simulink model "TSR_Scenario_003_cs"  (R2014b)
settings: Solver=ode5  SolverMode=SingleTasking  StartTime=0.0  StopTime=inf  FixedStep=1/100  RelTol=1e-3
PreLoadFcn:
  | mbxruntime.callbacks.PreLoadFcn(bdroot);
  | check_NUTS_defined;
  | 
  | assignin('base',['model_closed_' bdroot],false);
  | 
  | addpath('../includes_TSR/includes_TSR');
  | 
  | switch version('-release')
  | case {'2010a', '2010b', '2011a'}
  | addpath('../includes_TSR/ML2010b');
  | otherwise
  | addpath('../includes_TSR/ML2011b');
  | end
PostLoadFcn:
  | mbxruntime.callbacks.PostLoadFcn(bdroot);
InitFcn:
  | mbxruntime.callbacks.InitFcn(bdroot);
StartFcn:
  | mbxruntime.callbacks.StartFcn(bdroot);
StopFcn:
  | mbxruntime.callbacks.StopFcn(bdroot);
model workspace: external: MAT-File .\TSR_Scenario_003_cs_hws.mat (data not in the file)
undefined symbols (not defined in the file or in its folder): InitImageOutputDir, mbxruntime, OrientationPitch, OrientationRoll, PositionX, PositionY, PositionZ, tabledata, warningInitialVelocity, x0
undefined symbols (not defined in the file): SteeringColumn, SteeringWheel, TSR_Scenario_003_cs_031c08980fc50484, TSR_Scenario_003_cs_034f292ed02288d5, TSR_Scenario_003_cs_0459b3dfbc82c9a8, TSR_Scenario_003_cs_097620f815f21f1d, TSR_Scenario_003_cs_097d7573cc694bf5, TSR_Scenario_003_cs_0996a1a3dd5e2a3a, TSR_Scenario_003_cs_0f1849cdb4701326, TSR_Scenario_003_cs_10f4098912b3b5db, TSR_Scenario_003_cs_117f01ea831ec368, TSR_Scenario_003_cs_12cf78b79d36da1c, TSR_Scenario_003_cs_144fbb977118bf37, TSR_Scenario_003_cs_1523d5367c5052d0, TSR_Scenario_003_cs_1540f37e1ce5220e, TSR_Scenario_003_cs_15da4682074a9114, TSR_Scenario_003_cs_186e86d78e8adde8, TSR_Scenario_003_cs_198fefcb5c5d4c4a, TSR_Scenario_003_cs_1d24564a28ca8c57, TSR_Scenario_003_cs_1ea9b65b93b2d93e, TSR_Scenario_003_cs_1f4a4c0163bc654f, TSR_Scenario_003_cs_221c7f4f757b6f59, TSR_Scenario_003_cs_22229c9f69845439, TSR_Scenario_003_cs_230bf92302b3240a, TSR_Scenario_003_cs_23763ac742803108, TSR_Scenario_003_cs_237ee3c37f4d72b6, TSR_Scenario_003_cs_2956d712ba1268bc, TSR_Scenario_003_cs_2c8e6bdc42e74688, TSR_Scenario_003_cs_3037724928f99df0, TSR_Scenario_003_cs_31b44ca47ec5ff02, TSR_Scenario_003_cs_324745b613f45b9c, TSR_Scenario_003_cs_32b36e3fd4699b17, TSR_Scenario_003_cs_35d6077a5f3bdf8f, TSR_Scenario_003_cs_364710b5c901cafc, TSR_Scenario_003_cs_3727ee2f4430f2bb, TSR_Scenario_003_cs_382e41ab6806a13f, TSR_Scenario_003_cs_38ccddae174883be, TSR_Scenario_003_cs_3a0767dbf486e31b, TSR_Scenario_003_cs_3b460d19c10c747b, TSR_Scenario_003_cs_426c63b9f9c7abdf, TSR_Scenario_003_cs_42f1edf1b324bf4e, TSR_Scenario_003_cs_43b33e682c00a164, TSR_Scenario_003_cs_440a2f0d77aab01b, TSR_Scenario_003_cs_466378c5e179d625, TSR_Scenario_003_cs_4b8aa743d5bd8c1e, TSR_Scenario_003_cs_4bb095d5f4984042, TSR_Scenario_003_cs_4cec1a92176fe53d, TSR_Scenario_003_cs_4d6b6c843c52af2c, TSR_Scenario_003_cs_514fc139d324fd0d, TSR_Scenario_003_cs_51f4eff9e91179f9, TSR_Scenario_003_cs_56a9ea09cd860a89, TSR_Scenario_003_cs_5749c15298076949, TSR_Scenario_003_cs_576a8029b2a2792f, TSR_Scenario_003_cs_58b2f104991e8ca9, TSR_Scenario_003_cs_59a8a0af3bc025d5, TSR_Scenario_003_cs_5baf0e640050f43b, TSR_Scenario_003_cs_626299c795c4a86e, TSR_Scenario_003_cs_6499aa317499632d, TSR_Scenario_003_cs_676e881463a7df3e, TSR_Scenario_003_cs_68379cf1a8816ef6 ... (+115)
libraries: PreScanSimulinkLibrary x53, simulink_extras x37, simulink x29
(part 10 of 21)

== system TSR_Scenario_003_cs/Audi_A8_1/SteeringColumn_pivot_Mux ==
  X [m] : Inport
  Y [m] : Inport  Port=2
  Z [m] : Inport  Port=3
  Roll [rad] : Inport  Port=4
  Pitch [rad] : Inport  Port=5
  Yaw [rad] : Inport  Port=6
  Bus Creator : BusCreator  Inputs=3  OutDataTypeStr=Bus: PRESCAN_XYZ_DATA
  Bus Creator1 : BusCreator  Inputs=3  OutDataTypeStr=Bus: PRESCAN_RPY_DATA
  Bus Creator2 : BusCreator  Inputs=2  OutDataTypeStr=Bus: PRESCAN_POSE_DATA
  Joint : Outport
  wires:
  Yaw [rad]/1 -> Bus Creator1/3  "Yaw"
  Bus Creator1/1 -> Bus Creator2/2  "ORIENTATION"
  Bus Creator/1 -> Bus Creator2/1  "POSITION"
  X [m]/1 -> Bus Creator/1  "X"
  Y [m]/1 -> Bus Creator/2  "Y"
  Z [m]/1 -> Bus Creator/3  "Z"
  Bus Creator2/1 -> Joint/1
  Roll [rad]/1 -> Bus Creator1/1  "Roll"
  Pitch [rad]/1 -> Bus Creator1/2  "Pitch"

== system TSR_Scenario_003_cs/Audi_A8_1/SteeringWheel_pivot_Mux ==
  X [m] : Inport
  Y [m] : Inport  Port=2
  Z [m] : Inport  Port=3
  Roll [rad] : Inport  Port=4
  Pitch [rad] : Inport  Port=5
  Yaw [rad] : Inport  Port=6
  Bus Creator : BusCreator  Inputs=3  OutDataTypeStr=Bus: PRESCAN_XYZ_DATA
  Bus Creator1 : BusCreator  Inputs=3  OutDataTypeStr=Bus: PRESCAN_RPY_DATA
  Bus Creator2 : BusCreator  Inputs=2  OutDataTypeStr=Bus: PRESCAN_POSE_DATA
  Joint : Outport
  wires:
  Yaw [rad]/1 -> Bus Creator1/3  "Yaw"
  Bus Creator1/1 -> Bus Creator2/2  "ORIENTATION"
  Bus Creator/1 -> Bus Creator2/1  "POSITION"
  X [m]/1 -> Bus Creator/1  "X"
  Y [m]/1 -> Bus Creator/2  "Y"
  Z [m]/1 -> Bus Creator/3  "Z"
  Bus Creator2/1 -> Joint/1
  Roll [rad]/1 -> Bus Creator1/1  "Roll"
  Pitch [rad]/1 -> Bus Creator1/2  "Pitch"

== system TSR_Scenario_003_cs/Audi_A8_1/WheelDisplacement_Mux ==
  Steering Angle Front [rad] : Inport  Tag=inport/JointGroup  SampleTime=1/100  BusOutputAsStruct=on
  Steering Angle Rear [rad] : Inport  Tag=inport/JointGroup  Port=2  SampleTime=1/100  BusOutputAsStruct=on
  Rotation [rad] : Inport  Tag=inport/JointGroup  Port=3  SampleTime=1/100  BusOutputAsStruct=on
  zDisp FL [m] : Inport  Tag=inport/JointGroup  Port=4  SampleTime=1/100  BusOutputAsStruct=on
  zDisp FR [m] : Inport  Tag=inport/JointGroup  Port=5  SampleTime=1/100  BusOutputAsStruct=on
  zDisp RL [m] : Inport  Tag=inport/JointGroup  Port=6  SampleTime=1/100  BusOutputAsStruct=on
  zDisp RR [m] : Inport  Tag=inport/JointGroup  Port=7  SampleTime=1/100  BusOutputAsStruct=on
  Ground_{1..12} (12 alike) : Ground
  WheelL0_Mux : Subsystem  Tag=mux/Joint  mask(PreScan Mux Block){DisplayName=WheelL0}
      mask prompts: DisplayName "Display Name"
      mask help:
      | This block simulates a generic joint used for generic models. This joint can be enabled/disabled from the GUI.
      |
      | For more information, please click Help.
      settings: DeleteFcn=PreScanBlockDeleteFcn;
      mask Help: eval('openHelp(254)')
  WheelL1_Mux : Subsystem  Tag=mux/Joint  mask(PreScan Mux Block){DisplayName=WheelL1}
      mask prompts: DisplayName "Display Name"
      mask help:
      | This block simulates a generic joint used for generic models. This joint can be enabled/disabled from the GUI.
      |
      | For more information, please click Help.
      settings: DeleteFcn=PreScanBlockDeleteFcn;
      mask Help: eval('openHelp(254)')
  WheelR0_Mux : Subsystem  Tag=mux/Joint  mask(PreScan Mux Block){DisplayName=WheelR0}
      mask prompts: DisplayName "Display Name"
      mask help:
      | This block simulates a generic joint used for generic models. This joint can be enabled/disabled from the GUI.
      |
      | For more information, please click Help.
      settings: DeleteFcn=PreScanBlockDeleteFcn;
      mask Help: eval('openHelp(254)')
  WheelR1_Mux : Subsystem  Tag=mux/Joint  mask(PreScan Mux Block){DisplayName=WheelR1}
      mask prompts: DisplayName "Display Name"
      mask help:
      | This block simulates a generic joint used for generic models. This joint can be enabled/disabled from the GUI.
      |
      | For more information, please click Help.
      settings: DeleteFcn=PreScanBlockDeleteFcn;
      mask Help: eval('openHelp(254)')
  WheelL0_Audi_A8_1 : Outport  Tag=outport/JointActuator  OutDataTypeStr=Bus: PRESCAN_POSE_DATA  SampleTime=1/100
  WheelL1_Audi_A8_1 : Outport  Tag=outport/JointActuator  Port=2  OutDataTypeStr=Bus: PRESCAN_POSE_DATA  SampleTime=1/100
  WheelR0_Audi_A8_1 : Outport  Tag=outport/JointActuator  Port=3  OutDataTypeStr=Bus: PRESCAN_POSE_DATA  SampleTime=1/100
  WheelR1_Audi_A8_1 : Outport  Tag=outport/JointActuator  Port=4  OutDataTypeStr=Bus: PRESCAN_POSE_DATA  SampleTime=1/100
  wires:
  WheelL0_Mux/1(Joint) -> WheelL0_Audi_A8_1/1
  WheelL1_Mux/1(Joint) -> WheelL1_Audi_A8_1/1
  WheelR0_Mux/1(Joint) -> WheelR0_Audi_A8_1/1
  WheelR1_Mux/1(Joint) -> WheelR1_Audi_A8_1/1
  Steering Angle Front [rad]/1 -> WheelR0_Mux/6(Yaw [rad]), WheelL0_Mux/6(Yaw [rad])
  Steering Angle Rear [rad]/1 -> WheelR1_Mux/6(Yaw [rad]), WheelL1_Mux/6(Yaw [rad])
  Rotation [rad]/1 -> WheelR0_Mux/5(Pitch [rad]), WheelL0_Mux/5(Pitch [rad]), WheelR1_Mux/5(Pitch [rad]), WheelL1_Mux/5(Pitch [rad])
  zDisp FL [m]/1 -> WheelL0_Mux/3(Z [m])
  zDisp FR [m]/1 -> WheelR0_Mux/3(Z [m])
  zDisp RL [m]/1 -> WheelL1_Mux/3(Z [m])
  zDisp RR [m]/1 -> WheelR1_Mux/3(Z [m])
  Ground_1/1 -> WheelL0_Mux/1(X [m])
  Ground_2/1 -> WheelL0_Mux/2(Y [m])
  Ground_3/1 -> WheelL0_Mux/4(Roll [rad])
  Ground_4/1 -> WheelL1_Mux/1(X [m])
  Ground_5/1 -> WheelL1_Mux/2(Y [m])
  Ground_6/1 -> WheelL1_Mux/4(Roll [rad])
  Ground_7/1 -> WheelR0_Mux/1(X [m])
  Ground_8/1 -> WheelR0_Mux/2(Y [m])
  Ground_9/1 -> WheelR0_Mux/4(Roll [rad])
  Ground_10/1 -> WheelR1_Mux/1(X [m])
  Ground_11/1 -> WheelR1_Mux/2(Y [m])
  Ground_12/1 -> WheelR1_Mux/4(Roll [rad])

== system TSR_Scenario_003_cs/Audi_A8_1/d2r SteeringColumn_pivot_Mux ==
  Degrees in : Inport
  Gain1 : Gain  Gain=pi/180  SaturateOnIntegerOverflow=on  OutDataTypeStr=Inherit: Same as input  ParamDataTypeStr=Inherit: Same as input
  Radians out : Outport  InitialOutput=0
  wires:
  Gain1/1 -> Radians out/1
  Degrees in/1 -> Gain1/1

== system TSR_Scenario_003_cs/Audi_A8_1/d2r SteeringWheel_pivot_Mux ==
  Degrees in : Inport
  Gain1 : Gain  Gain=pi/180  SaturateOnIntegerOverflow=on  OutDataTypeStr=Inherit: Same as input  ParamDataTypeStr=Inherit: Same as input
  Radians out : Outport  InitialOutput=0
  wires:
  Gain1/1 -> Radians out/1
  Degrees in/1 -> Gain1/1

== system TSR_Scenario_003_cs/Audi_A8_1/d2r WheelDisplacement_Mux 1 ==
  Degrees in : Inport
  Gain1 : Gain  Gain=pi/180  SaturateOnIntegerOverflow=on  OutDataTypeStr=Inherit: Same as input  ParamDataTypeStr=Inherit: Same as input
  Radians out : Outport  InitialOutput=0
  wires:
  Gain1/1 -> Radians out/1
  Degrees in/1 -> Gain1/1

== system TSR_Scenario_003_cs/BMW_X5_1/Dynamics_Empty ==
  note: For state mode 'Dynamic' positions
      | are not taken into account, as they
      | are computed by integrating velocity.
      | Click annotation for Help.
  note: For state mode 'Dynamic' positions
      | are not taken into account, as they
      | are computed by integrating velocity.
      | Click annotation for Help.
  Ground_{1..9} (9 alike) : Ground
  MuxState : Subsystem  Tag=mux/State  mask(Empty Dynamics State Block){positioningmode=on, TimeStep=1/100}
      mask prompts: positioningmode "Positioning Mode"; TimeStep "Auto Assigned: Time Step [s]"
      mask help:
      | Build the state of an actor based on user input.
      | The user can either use positioning mode or dynamics mode.
      | - When using positioning mode the position and orientation of the actor are set directly based on the input. Expected input is relative to the initial position and orientation of the actor. It's also possible to specify the velocity of the actor, though this input isn't used, only passed on.
      | - When using dynamics mode the position input is ignored. Expected input is velocity and orientation. The velocity is relative the current orientation of the actor, while orientation is relative to its initial orientation. The position of the actor is calculated based on the velocity and orientation given.
      settings: DeleteFcn=PreScanBlockDeleteFcn;
  STATE_BMW_X5_1 : Subsystem  Tag=mux/StatePort  Priority=0  LoadFcn=load PrescanStateActuatorData  mask(PreScan Sink Block: State){x0=TSR_Scenario_003_cs_BMW_X5_1_Dynamics_Empty_STATE_BMW_X5_1_x0, y0=TSR_Scenario_003_cs_BMW_X5_1_Dynamics_Empty_STATE_BMW_X5_1_y0, z0=TSR_Scenario_003_cs_BMW_X5_1_Dynamics_Empty_STATE_BMW_X5_1_z0, Roll0=TSR_Scenario_003_cs_15da4682074a9114, Pitch0=TSR_Scenario_003_cs_d01058e0ce79997b, Yaw0=TSR_Scenario_003_cs_BMW_X5_1_Dynamics_Empty_STATE_BMW_X5_1_Yaw0, TimeStep=1/100}
      mask prompts: x0 "Ini x-position VEHICLE wrt GLOBAL axis system [m]"; y0 "Ini y-position VEHICLE wrt GLOBAL axis system [m]"; z0 "Ini z-position VEHICLE wrt GLOBAL axis system [m]"; Roll0 "Ini roll-angle BODY wrt VEHICLE axis system [deg]"; Pitch0 "Ini pitch-angle BODY wrt VEHICLE axis system [deg]"; Yaw0 "Ini yaw-angle VEHICLE wrt GLOBAL axis system [deg]"; TimeStep "Auto-Assigned: Upload Period [s]"
      mask help:
      | The Actor State contains a vector signal of size (9x1), containing the following signals:
      |
      | -  Position                  (x,y,z)                                     [m]
      | -  Velocity                  (vx,vy,vz)                               [m/s]
      | -  Angles                    (Roll, Pitch, Yaw)                   [rad]
      |
      | The Actor state is defined in the global axis system.
      | The state is superponed on the Initial position defined in the GUI.
      |
      | For more information, please click Help.
      settings: DeleteFcn=PreScanBlockDeleteFcn;
      mask Help: eval('openHelp(222)')
      mask Display: image(imread('State.png'))
  State : Outport  Tag=outport/StateOutport  SampleTime=1/100
  wires:
  STATE_BMW_X5_1/1(StateBus) -> State/1
  MuxState/1(state) -> STATE_BMW_X5_1/1(State)
  Ground_1/1 -> MuxState/1(x [m])
  Ground_2/1 -> MuxState/2(y [m])
  Ground_3/1 -> MuxState/3(z [m])
  Ground_4/1 -> MuxState/4(dx [m/s])
  Ground_5/1 -> MuxState/5(dy [m/s])
  Ground_6/1 -> MuxState/6(dz [m/s])
  Ground_7/1 -> MuxState/7(R [rad])
  Ground_8/1 -> MuxState/8(P [rad])
  Ground_9/1 -> MuxState/9(Y [rad])

== system TSR_Scenario_003_cs/BMW_X5_1/SELF_Demux ==
  SELF : Inport  OutDataTypeStr=Bus: PRESCAN_SELFSENSORDATA
  Bus Selector : BusSelector  OutputSignals=PositionX,PositionY,PositionZ,OrientationRoll,OrientationPitch,OrientationYaw,Velocity,Yaw_rate,Lat,Long,Alt
  Demux2 : Demux  Outputs=3
  Gain : Gain  Gain=180/pi
  Gain1 : Gain  Gain=180/pi
  Vector Concatenate1 : Concatenate  NumInputs=3
  compas converter : Subsystem
  x [m] : Outport
  y [m] : Outport  Port=2
  z [m] : Outport  Port=3
  rotx [deg] : Outport  Port=4
  roty [deg] : Outport  Port=5
  rotz [deg] : Outport  Port=6
  GPS lat [deg] : Outport  Port=7
  GPS long [deg] : Outport  Port=8
  GPS alt [m] : Outport  Port=9
  velocity [m/s] : Outport  Port=10
  heading [deg] : Outport  Port=11
  yaw rate [deg/s] : Outport  Port=12
  wires:
  Bus Selector/11 -> GPS alt [m]/1  "<Alt>"
  Bus Selector/10 -> GPS long [deg]/1  "<Long>"
  Bus Selector/9 -> GPS lat [deg]/1  "<Lat>"
  Bus Selector/8 -> Gain1/1  "<Yaw_rate>"
  Bus Selector/7 -> velocity [m/s]/1  "<Velocity>"
  Bus Selector/6 -> compas converter/1(rotz [rad]), Vector Concatenate1/3  "<OrientationYaw>"
  Bus Selector/5 -> Vector Concatenate1/2  "<OrientationPitch>"
  Bus Selector/4 -> Vector Concatenate1/1  "<OrientationRoll>"
  Vector Concatenate1/1 -> Gain/1
  Bus Selector/3 -> z [m]/1  "<PositionZ>"
  Bus Selector/2 -> y [m]/1  "<PositionY>"
  Bus Selector/1 -> x [m]/1  "<PositionX>"
  SELF/1 -> Bus Selector/1
  Gain/1 -> Demux2/1
  Demux2/1 -> rotx [deg]/1
  Demux2/2 -> roty [deg]/1
  Demux2/3 -> rotz [deg]/1
  compas converter/1(heading [deg]) -> heading [deg]/1
  Gain1/1 -> yaw rate [deg/s]/1

== system TSR_Scenario_003_cs/BMW_X5_2/Dynamics_Empty ==
  note: For state mode 'Dynamic' positions
      | are not taken into account, as they
      | are computed by integrating velocity.
      | Click annotation for Help.
  note: For state mode 'Dynamic' positions
      | are not taken into account, as they
      | are computed by integrating velocity.
      | Click annotation for Help.
  Ground_{1..9} (9 alike) : Ground
  MuxState : Subsystem  Tag=mux/State  mask(Empty Dynamics State Block){positioningmode=on, TimeStep=1/100}
      mask prompts: positioningmode "Positioning Mode"; TimeStep "Auto Assigned: Time Step [s]"
      mask help:
      | Build the state of an actor based on user input.
      | The user can either use positioning mode or dynamics mode.
      | - When using positioning mode the position and orientation of the actor are set directly based on the input. Expected input is relative to the initial position and orientation of the actor. It's also possible to specify the velocity of the actor, though this input isn't used, only passed on.
      | - When using dynamics mode the position input is ignored. Expected input is velocity and orientation. The velocity is relative the current orientation of the actor, while orientation is relative to its initial orientation. The position of the actor is calculated based on the velocity and orientation given.
      settings: DeleteFcn=PreScanBlockDeleteFcn;
  STATE_BMW_X5_2 : Subsystem  Tag=mux/StatePort  Priority=0  LoadFcn=load PrescanStateActuatorData  mask(PreScan Sink Block: State){x0=TSR_Scenario_003_cs_BMW_X5_2_Dynamics_Empty_STATE_BMW_X5_2_x0, y0=TSR_Scenario_003_cs_BMW_X5_2_Dynamics_Empty_STATE_BMW_X5_2_y0, z0=TSR_Scenario_003_cs_BMW_X5_2_Dynamics_Empty_STATE_BMW_X5_2_z0, Roll0=TSR_Scenario_003_cs_683e8ba4a0f8240e, Pitch0=TSR_Scenario_003_cs_bee4b2d4b9008bb0, Yaw0=TSR_Scenario_003_cs_BMW_X5_2_Dynamics_Empty_STATE_BMW_X5_2_Yaw0, TimeStep=1/100}
      mask prompts: x0 "Ini x-position VEHICLE wrt GLOBAL axis system [m]"; y0 "Ini y-position VEHICLE wrt GLOBAL axis system [m]"; z0 "Ini z-position VEHICLE wrt GLOBAL axis system [m]"; Roll0 "Ini roll-angle BODY wrt VEHICLE axis system [deg]"; Pitch0 "Ini pitch-angle BODY wrt VEHICLE axis system [deg]"; Yaw0 "Ini yaw-angle VEHICLE wrt GLOBAL axis system [deg]"; TimeStep "Auto-Assigned: Upload Period [s]"
      mask help:
      | The Actor State contains a vector signal of size (9x1), containing the following signals:
      |
      | -  Position                  (x,y,z)                                     [m]
      | -  Velocity                  (vx,vy,vz)                               [m/s]
      | -  Angles                    (Roll, Pitch, Yaw)                   [rad]
      |
      | The Actor state is defined in the global axis system.
      | The state is superponed on the Initial position defined in the GUI.
      |
      | For more information, please click Help.
      settings: DeleteFcn=PreScanBlockDeleteFcn;
      mask Help: eval('openHelp(222)')
      mask Display: image(imread('State.png'))
  State : Outport  Tag=outport/StateOutport  SampleTime=1/100
  wires:
  STATE_BMW_X5_2/1(StateBus) -> State/1
  MuxState/1(state) -> STATE_BMW_X5_2/1(State)
  Ground_1/1 -> MuxState/1(x [m])
  Ground_2/1 -> MuxState/2(y [m])
  Ground_3/1 -> MuxState/3(z [m])
  Ground_4/1 -> MuxState/4(dx [m/s])
  Ground_5/1 -> MuxState/5(dy [m/s])
  Ground_6/1 -> MuxState/6(dz [m/s])
  Ground_7/1 -> MuxState/7(R [rad])
  Ground_8/1 -> MuxState/8(P [rad])
  Ground_9/1 -> MuxState/9(Y [rad])

== system TSR_Scenario_003_cs/BMW_X5_2/SELF_Demux ==
  SELF : Inport  OutDataTypeStr=Bus: PRESCAN_SELFSENSORDATA
  Bus Selector : BusSelector  OutputSignals=PositionX,PositionY,PositionZ,OrientationRoll,OrientationPitch,OrientationYaw,Velocity,Yaw_rate,Lat,Long,Alt
  Demux2 : Demux  Outputs=3
  Gain : Gain  Gain=180/pi
  Gain1 : Gain  Gain=180/pi
  Vector Concatenate1 : Concatenate  NumInputs=3
  compas converter : Subsystem
  x [m] : Outport
  y [m] : Outport  Port=2
  z [m] : Outport  Port=3
  rotx [deg] : Outport  Port=4
  roty [deg] : Outport  Port=5
  rotz [deg] : Outport  Port=6
  GPS lat [deg] : Outport  Port=7
  GPS long [deg] : Outport  Port=8
  GPS alt [m] : Outport  Port=9
  velocity [m/s] : Outport  Port=10
  heading [deg] : Outport  Port=11
  yaw rate [deg/s] : Outport  Port=12
  wires:
  Bus Selector/11 -> GPS alt [m]/1  "<Alt>"
  Bus Selector/10 -> GPS long [deg]/1  "<Long>"
  Bus Selector/9 -> GPS lat [deg]/1  "<Lat>"
  Bus Selector/8 -> Gain1/1  "<Yaw_rate>"
  Bus Selector/7 -> velocity [m/s]/1  "<Velocity>"
  Bus Selector/6 -> compas converter/1(rotz [rad]), Vector Concatenate1/3  "<OrientationYaw>"
  Bus Selector/5 -> Vector Concatenate1/2  "<OrientationPitch>"
  Bus Selector/4 -> Vector Concatenate1/1  "<OrientationRoll>"
  Vector Concatenate1/1 -> Gain/1
  Bus Selector/3 -> z [m]/1  "<PositionZ>"
  Bus Selector/2 -> y [m]/1  "<PositionY>"
  Bus Selector/1 -> x [m]/1  "<PositionX>"
  SELF/1 -> Bus Selector/1
  Gain/1 -> Demux2/1
  Demux2/1 -> rotx [deg]/1
  Demux2/2 -> roty [deg]/1
  Demux2/3 -> rotz [deg]/1
  compas converter/1(heading [deg]) -> heading [deg]/1
  Gain1/1 -> yaw rate [deg/s]/1

== system TSR_Scenario_003_cs/BMW_X5_3/Dynamics_Empty ==
  note: For state mode 'Dynamic' positions
      | are not taken into account, as they
      | are computed by integrating velocity.
      | Click annotation for Help.
  note: For state mode 'Dynamic' positions
      | are not taken into account, as they
      | are computed by integrating velocity.
      | Click annotation for Help.
  Ground_{1..9} (9 alike) : Ground
  MuxState : Subsystem  Tag=mux/State  mask(Empty Dynamics State Block){positioningmode=on, TimeStep=1/100}
      mask prompts: positioningmode "Positioning Mode"; TimeStep "Auto Assigned: Time Step [s]"
      mask help:
      | Build the state of an actor based on user input.
      | The user can either use positioning mode or dynamics mode.
      | - When using positioning mode the position and orientation of the actor are set directly based on the input. Expected input is relative to the initial position and orientation of the actor. It's also possible to specify the velocity of the actor, though this input isn't used, only passed on.
      | - When using dynamics mode the position input is ignored. Expected input is velocity and orientation. The velocity is relative the current orientation of the actor, while orientation is relative to its initial orientation. The position of the actor is calculated based on the velocity and orientation given.
      settings: DeleteFcn=PreScanBlockDeleteFcn;
  STATE_BMW_X5_3 : Subsystem  Tag=mux/StatePort  Priority=0  LoadFcn=load PrescanStateActuatorData  mask(PreScan Sink Block: State){x0=TSR_Scenario_003_cs_BMW_X5_3_Dynamics_Empty_STATE_BMW_X5_3_x0, y0=TSR_Scenario_003_cs_BMW_X5_3_Dynamics_Empty_STATE_BMW_X5_3_y0, z0=TSR_Scenario_003_cs_BMW_X5_3_Dynamics_Empty_STATE_BMW_X5_3_z0, Roll0=TSR_Scenario_003_cs_b1ad55d7788b6684, Pitch0=TSR_Scenario_003_cs_7e63232506427d45, Yaw0=TSR_Scenario_003_cs_BMW_X5_3_Dynamics_Empty_STATE_BMW_X5_3_Yaw0, TimeStep=1/100}
      mask prompts: x0 "Ini x-position VEHICLE wrt GLOBAL axis system [m]"; y0 "Ini y-position VEHICLE wrt GLOBAL axis system [m]"; z0 "Ini z-position VEHICLE wrt GLOBAL axis system [m]"; Roll0 "Ini roll-angle BODY wrt VEHICLE axis system [deg]"; Pitch0 "Ini pitch-angle BODY wrt VEHICLE axis system [deg]"; Yaw0 "Ini yaw-angle VEHICLE wrt GLOBAL axis system [deg]"; TimeStep "Auto-Assigned: Upload Period [s]"
      mask help:
      | The Actor State contains a vector signal of size (9x1), containing the following signals:
      |
      | -  Position                  (x,y,z)                                     [m]
      | -  Velocity                  (vx,vy,vz)                               [m/s]
      | -  Angles                    (Roll, Pitch, Yaw)                   [rad]
      |
      | The Actor state is defined in the global axis system.
      | The state is superponed on the Initial position defined in the GUI.
      |
      | For more information, please click Help.
      settings: DeleteFcn=PreScanBlockDeleteFcn;
      mask Help: eval('openHelp(222)')
      mask Display: image(imread('State.png'))
  State : Outport  Tag=outport/StateOutport  SampleTime=1/100
  wires:
  STATE_BMW_X5_3/1(StateBus) -> State/1
  MuxState/1(state) -> STATE_BMW_X5_3/1(State)
  Ground_1/1 -> MuxState/1(x [m])
  Ground_2/1 -> MuxState/2(y [m])
  Ground_3/1 -> MuxState/3(z [m])
  Ground_4/1 -> MuxState/4(dx [m/s])
  Ground_5/1 -> MuxState/5(dy [m/s])
  Ground_6/1 -> MuxState/6(dz [m/s])
  Ground_7/1 -> MuxState/7(R [rad])
  Ground_8/1 -> MuxState/8(P [rad])
  Ground_9/1 -> MuxState/9(Y [rad])

== system TSR_Scenario_003_cs/BMW_X5_3/SELF_Demux ==
  SELF : Inport  OutDataTypeStr=Bus: PRESCAN_SELFSENSORDATA
  Bus Selector : BusSelector  OutputSignals=PositionX,PositionY,PositionZ,OrientationRoll,OrientationPitch,OrientationYaw,Velocity,Yaw_rate,Lat,Long,Alt
  Demux2 : Demux  Outputs=3
  Gain : Gain  Gain=180/pi
  Gain1 : Gain  Gain=180/pi
  Vector Concatenate1 : Concatenate  NumInputs=3
  compas converter : Subsystem
  x [m] : Outport
  y [m] : Outport  Port=2
  z [m] : Outport  Port=3
  rotx [deg] : Outport  Port=4
  roty [deg] : Outport  Port=5
  rotz [deg] : Outport  Port=6
  GPS lat [deg] : Outport  Port=7
  GPS long [deg] : Outport  Port=8
  GPS alt [m] : Outport  Port=9
  velocity [m/s] : Outport  Port=10
  heading [deg] : Outport  Port=11
  yaw rate [deg/s] : Outport  Port=12
  wires:
  Bus Selector/11 -> GPS alt [m]/1  "<Alt>"
  Bus Selector/10 -> GPS long [deg]/1  "<Long>"
  Bus Selector/9 -> GPS lat [deg]/1  "<Lat>"
  Bus Selector/8 -> Gain1/1  "<Yaw_rate>"
  Bus Selector/7 -> velocity [m/s]/1  "<Velocity>"
  Bus Selector/6 -> compas converter/1(rotz [rad]), Vector Concatenate1/3  "<OrientationYaw>"
  Bus Selector/5 -> Vector Concatenate1/2  "<OrientationPitch>"
  Bus Selector/4 -> Vector Concatenate1/1  "<OrientationRoll>"
  Vector Concatenate1/1 -> Gain/1
  Bus Selector/3 -> z [m]/1  "<PositionZ>"
  Bus Selector/2 -> y [m]/1  "<PositionY>"
  Bus Selector/1 -> x [m]/1  "<PositionX>"
  SELF/1 -> Bus Selector/1
  Gain/1 -> Demux2/1
  Demux2/1 -> rotx [deg]/1
  Demux2/2 -> roty [deg]/1
  Demux2/3 -> rotz [deg]/1
  compas converter/1(heading [deg]) -> heading [deg]/1
  Gain1/1 -> yaw rate [deg/s]/1

== system TSR_Scenario_003_cs/BMW_Z3_1/Dynamics_Empty ==
  note: For state mode 'Dynamic' positions
      | are not taken into account, as they
      | are computed by integrating velocity.
      | Click annotation for Help.
  note: For state mode 'Dynamic' positions
      | are not taken into account, as they
      | are computed by integrating velocity.
      | Click annotation for Help.
  Ground_{1..9} (9 alike) : Ground
  MuxState : Subsystem  Tag=mux/State  mask(Empty Dynamics State Block){positioningmode=on, TimeStep=1/100}
      mask prompts: positioningmode "Positioning Mode"; TimeStep "Auto Assigned: Time Step [s]"
      mask help:
      | Build the state of an actor based on user input.
      | The user can either use positioning mode or dynamics mode.
      | - When using positioning mode the position and orientation of the actor are set directly based on the input. Expected input is relative to the initial position and orientation of the actor. It's also possible to specify the velocity of the actor, though this input isn't used, only passed on.
      | - When using dynamics mode the position input is ignored. Expected input is velocity and orientation. The velocity is relative the current orientation of the actor, while orientation is relative to its initial orientation. The position of the actor is calculated based on the velocity and orientation given.
      settings: DeleteFcn=PreScanBlockDeleteFcn;
  STATE_BMW_Z3_1 : Subsystem  Tag=mux/StatePort  Priority=0  LoadFcn=load PrescanStateActuatorData  mask(PreScan Sink Block: State){x0=TSR_Scenario_003_cs_BMW_Z3_1_Dynamics_Empty_STATE_BMW_Z3_1_x0, y0=TSR_Scenario_003_cs_BMW_Z3_1_Dynamics_Empty_STATE_BMW_Z3_1_y0, z0=TSR_Scenario_003_cs_BMW_Z3_1_Dynamics_Empty_STATE_BMW_Z3_1_z0, Roll0=TSR_Scenario_003_cs_83f6319363c4fbdc, Pitch0=TSR_Scenario_003_cs_dd58b79918ad8b87, Yaw0=TSR_Scenario_003_cs_BMW_Z3_1_Dynamics_Empty_STATE_BMW_Z3_1_Yaw0, TimeStep=1/100}
      mask prompts: x0 "Ini x-position VEHICLE wrt GLOBAL axis system [m]"; y0 "Ini y-position VEHICLE wrt GLOBAL axis system [m]"; z0 "Ini z-position VEHICLE wrt GLOBAL axis system [m]"; Roll0 "Ini roll-angle BODY wrt VEHICLE axis system [deg]"; Pitch0 "Ini pitch-angle BODY wrt VEHICLE axis system [deg]"; Yaw0 "Ini yaw-angle VEHICLE wrt GLOBAL axis system [deg]"; TimeStep "Auto-Assigned: Upload Period [s]"
      mask help:
      | The Actor State contains a vector signal of size (9x1), containing the following signals:
      |
      | -  Position                  (x,y,z)                                     [m]
      | -  Velocity                  (vx,vy,vz)                               [m/s]
      | -  Angles                    (Roll, Pitch, Yaw)                   [rad]
      |
      | The Actor state is defined in the global axis system.
      | The state is superponed on the Initial position defined in the GUI.
      |
      | For more information, please click Help.
      settings: DeleteFcn=PreScanBlockDeleteFcn;
      mask Help: eval('openHelp(222)')
      mask Display: image(imread('State.png'))
  State : Outport  Tag=outport/StateOutport  SampleTime=1/100
  wires:
  STATE_BMW_Z3_1/1(StateBus) -> State/1
  MuxState/1(state) -> STATE_BMW_Z3_1/1(State)
  Ground_1/1 -> MuxState/1(x [m])
  Ground_2/1 -> MuxState/2(y [m])
  Ground_3/1 -> MuxState/3(z [m])
  Ground_4/1 -> MuxState/4(dx [m/s])
  Ground_5/1 -> MuxState/5(dy [m/s])
  Ground_6/1 -> MuxState/6(dz [m/s])
  Ground_7/1 -> MuxState/7(R [rad])
  Ground_8/1 -> MuxState/8(P [rad])
  Ground_9/1 -> MuxState/9(Y [rad])

== system TSR_Scenario_003_cs/BMW_Z3_1/SELF_Demux ==
  SELF : Inport  OutDataTypeStr=Bus: PRESCAN_SELFSENSORDATA
  Bus Selector : BusSelector  OutputSignals=PositionX,PositionY,PositionZ,OrientationRoll,OrientationPitch,OrientationYaw,Velocity,Yaw_rate,Lat,Long,Alt
  Demux2 : Demux  Outputs=3
  Gain : Gain  Gain=180/pi
  Gain1 : Gain  Gain=180/pi
  Vector Concatenate1 : Concatenate  NumInputs=3
  compas converter : Subsystem
  x [m] : Outport
  y [m] : Outport  Port=2
  z [m] : Outport  Port=3
  rotx [deg] : Outport  Port=4
  roty [deg] : Outport  Port=5
  rotz [deg] : Outport  Port=6
  GPS lat [deg] : Outport  Port=7
  GPS long [deg] : Outport  Port=8
  GPS alt [m] : Outport  Port=9
  velocity [m/s] : Outport  Port=10
  heading [deg] : Outport  Port=11
  yaw rate [deg/s] : Outport  Port=12
  wires:
  Bus Selector/11 -> GPS alt [m]/1  "<Alt>"
  Bus Selector/10 -> GPS long [deg]/1  "<Long>"
  Bus Selector/9 -> GPS lat [deg]/1  "<Lat>"
  Bus Selector/8 -> Gain1/1  "<Yaw_rate>"
  Bus Selector/7 -> velocity [m/s]/1  "<Velocity>"
  Bus Selector/6 -> compas converter/1(rotz [rad]), Vector Concatenate1/3  "<OrientationYaw>"
  Bus Selector/5 -> Vector Concatenate1/2  "<OrientationPitch>"
  Bus Selector/4 -> Vector Concatenate1/1  "<OrientationRoll>"
  Vector Concatenate1/1 -> Gain/1
  Bus Selector/3 -> z [m]/1  "<PositionZ>"
  Bus Selector/2 -> y [m]/1  "<PositionY>"
  Bus Selector/1 -> x [m]/1  "<PositionX>"
  SELF/1 -> Bus Selector/1
  Gain/1 -> Demux2/1
  Demux2/1 -> rotx [deg]/1
  Demux2/2 -> roty [deg]/1
  Demux2/3 -> rotz [deg]/1
  compas converter/1(heading [deg]) -> heading [deg]/1
  Gain1/1 -> yaw rate [deg/s]/1

== system TSR_Scenario_003_cs/Citroen_C3_1/Dynamics_Empty ==
  note: For state mode 'Dynamic' positions
      | are not taken into account, as they
      | are computed by integrating velocity.
      | Click annotation for Help.
  note: For state mode 'Dynamic' positions
      | are not taken into account, as they
      | are computed by integrating velocity.
      | Click annotation for Help.
  Ground_{1..9} (9 alike) : Ground
  MuxState : Subsystem  Tag=mux/State  mask(Empty Dynamics State Block){positioningmode=on, TimeStep=1/100}
      mask prompts: positioningmode "Positioning Mode"; TimeStep "Auto Assigned: Time Step [s]"
      mask help:
      | Build the state of an actor based on user input.
      | The user can either use positioning mode or dynamics mode.
      | - When using positioning mode the position and orientation of the actor are set directly based on the input. Expected input is relative to the initial position and orientation of the actor. It's also possible to specify the velocity of the actor, though this input isn't used, only passed on.
      | - When using dynamics mode the position input is ignored. Expected input is velocity and orientation. The velocity is relative the current orientation of the actor, while orientation is relative to its initial orientation. The position of the actor is calculated based on the velocity and orientation given.
      settings: DeleteFcn=PreScanBlockDeleteFcn;
  STATE_Citroen_C3_1 : Subsystem  Tag=mux/StatePort  Priority=0  LoadFcn=load PrescanStateActuatorData  mask(PreScan Sink Block: State){x0=TSR_Scenario_003_cs_034f292ed02288d5, y0=TSR_Scenario_003_cs_186e86d78e8adde8, z0=TSR_Scenario_003_cs_4b8aa743d5bd8c1e, Roll0=TSR_Scenario_003_cs_8267bd55a7ad8317, Pitch0=TSR_Scenario_003_cs_e6d6ad001b944fd2, Yaw0=TSR_Scenario_003_cs_7873a486ae681bd2, TimeStep=1/100}
      mask prompts: x0 "Ini x-position VEHICLE wrt GLOBAL axis system [m]"; y0 "Ini y-position VEHICLE wrt GLOBAL axis system [m]"; z0 "Ini z-position VEHICLE wrt GLOBAL axis system [m]"; Roll0 "Ini roll-angle BODY wrt VEHICLE axis system [deg]"; Pitch0 "Ini pitch-angle BODY wrt VEHICLE axis system [deg]"; Yaw0 "Ini yaw-angle VEHICLE wrt GLOBAL axis system [deg]"; TimeStep "Auto-Assigned: Upload Period [s]"
      mask help:
      | The Actor State contains a vector signal of size (9x1), containing the following signals:
      |
      | -  Position                  (x,y,z)                                     [m]
      | -  Velocity                  (vx,vy,vz)                               [m/s]
      | -  Angles                    (Roll, Pitch, Yaw)                   [rad]
      |
      | The Actor state is defined in the global axis system.
      | The state is superponed on the Initial position defined in the GUI.
      |
      | For more information, please click Help.
      settings: DeleteFcn=PreScanBlockDeleteFcn;
      mask Help: eval('openHelp(222)')
      mask Display: image(imread('State.png'))
  State : Outport  Tag=outport/StateOutport  SampleTime=1/100
  wires:
  STATE_Citroen_C3_1/1(StateBus) -> State/1
  MuxState/1(state) -> STATE_Citroen_C3_1/1(State)
  Ground_1/1 -> MuxState/1(x [m])
  Ground_2/1 -> MuxState/2(y [m])
  Ground_3/1 -> MuxState/3(z [m])
  Ground_4/1 -> MuxState/4(dx [m/s])
  Ground_5/1 -> MuxState/5(dy [m/s])
  Ground_6/1 -> MuxState/6(dz [m/s])
  Ground_7/1 -> MuxState/7(R [rad])
  Ground_8/1 -> MuxState/8(P [rad])
  Ground_9/1 -> MuxState/9(Y [rad])

== system TSR_Scenario_003_cs/Citroen_C3_1/SELF_Demux ==
  SELF : Inport  OutDataTypeStr=Bus: PRESCAN_SELFSENSORDATA
  Bus Selector : BusSelector  OutputSignals=PositionX,PositionY,PositionZ,OrientationRoll,OrientationPitch,OrientationYaw,Velocity,Yaw_rate,Lat,Long,Alt
  Demux2 : Demux  Outputs=3
  Gain : Gain  Gain=180/pi
  Gain1 : Gain  Gain=180/pi
  Vector Concatenate1 : Concatenate  NumInputs=3
  compas converter : Subsystem
  x [m] : Outport
  y [m] : Outport  Port=2
  z [m] : Outport  Port=3
  rotx [deg] : Outport  Port=4
  roty [deg] : Outport  Port=5
  rotz [deg] : Outport  Port=6
  GPS lat [deg] : Outport  Port=7
  GPS long [deg] : Outport  Port=8
  GPS alt [m] : Outport  Port=9
  velocity [m/s] : Outport  Port=10
  heading [deg] : Outport  Port=11
  yaw rate [deg/s] : Outport  Port=12
  wires:
  Bus Selector/11 -> GPS alt [m]/1  "<Alt>"
  Bus Selector/10 -> GPS long [deg]/1  "<Long>"
  Bus Selector/9 -> GPS lat [deg]/1  "<Lat>"
  Bus Selector/8 -> Gain1/1  "<Yaw_rate>"
  Bus Selector/7 -> velocity [m/s]/1  "<Velocity>"
  Bus Selector/6 -> compas converter/1(rotz [rad]), Vector Concatenate1/3  "<OrientationYaw>"
  Bus Selector/5 -> Vector Concatenate1/2  "<OrientationPitch>"
  Bus Selector/4 -> Vector Concatenate1/1  "<OrientationRoll>"
  Vector Concatenate1/1 -> Gain/1
  Bus Selector/3 -> z [m]/1  "<PositionZ>"
  Bus Selector/2 -> y [m]/1  "<PositionY>"
  Bus Selector/1 -> x [m]/1  "<PositionX>"
  SELF/1 -> Bus Selector/1
  Gain/1 -> Demux2/1
  Demux2/1 -> rotx [deg]/1
  Demux2/2 -> roty [deg]/1
  Demux2/3 -> rotz [deg]/1
  compas converter/1(heading [deg]) -> heading [deg]/1
  Gain1/1 -> yaw rate [deg/s]/1

== system TSR_Scenario_003_cs/Daf_95_1/SELF_Demux ==
  SELF : Inport  OutDataTypeStr=Bus: PRESCAN_SELFSENSORDATA
  Bus Selector : BusSelector  OutputSignals=PositionX,PositionY,PositionZ,OrientationRoll,OrientationPitch,OrientationYaw,Velocity,Yaw_rate,Lat,Long,Alt
  Demux2 : Demux  Outputs=3
  Gain : Gain  Gain=180/pi
  Gain1 : Gain  Gain=180/pi
  Vector Concatenate1 : Concatenate  NumInputs=3
  compas converter : Subsystem
  x [m] : Outport
  y [m] : Outport  Port=2
  z [m] : Outport  Port=3
  rotx [deg] : Outport  Port=4
  roty [deg] : Outport  Port=5
  rotz [deg] : Outport  Port=6
  GPS lat [deg] : Outport  Port=7
  GPS long [deg] : Outport  Port=8
  GPS alt [m] : Outport  Port=9
  velocity [m/s] : Outport  Port=10
  heading [deg] : Outport  Port=11
  yaw rate [deg/s] : Outport  Port=12
  wires:
  Bus Selector/11 -> GPS alt [m]/1  "<Alt>"
  Bus Selector/10 -> GPS long [deg]/1  "<Long>"
  Bus Selector/9 -> GPS lat [deg]/1  "<Lat>"
  Bus Selector/8 -> Gain1/1  "<Yaw_rate>"
  Bus Selector/7 -> velocity [m/s]/1  "<Velocity>"
  Bus Selector/6 -> compas converter/1(rotz [rad]), Vector Concatenate1/3  "<OrientationYaw>"
  Bus Selector/5 -> Vector Concatenate1/2  "<OrientationPitch>"
  Bus Selector/4 -> Vector Concatenate1/1  "<OrientationRoll>"
  Vector Concatenate1/1 -> Gain/1
  Bus Selector/3 -> z [m]/1  "<PositionZ>"
  Bus Selector/2 -> y [m]/1  "<PositionY>"
  Bus Selector/1 -> x [m]/1  "<PositionX>"
  SELF/1 -> Bus Selector/1
  Gain/1 -> Demux2/1
  Demux2/1 -> rotx [deg]/1
  Demux2/2 -> roty [deg]/1
  Demux2/3 -> rotz [deg]/1
  compas converter/1(heading [deg]) -> heading [deg]/1
  Gain1/1 -> yaw rate [deg/s]/1

== system TSR_Scenario_003_cs/Female_RegularAni_1/Animation ==
  In1 : Inport
  Bus Creator : BusCreator  Inputs=2  OutDataTypeStr=Bus: PRESCAN_ANIMACTUATORDATA  NonVirtualBus=on
  Bus Selector : BusSelector  OutputSignals=VelocityX,VelocityY,VelocityZ
  Data Type Conversion : DataTypeConversion  OutDataTypeStr=int32
  Mux : Mux  Inputs=3
  Product : Product  RndMeth=Zero
  RunningScale : Constant  Value=RunningScale
  Switch : Switch  Threshold=2
  WalkingScale : Constant  Value=WalkingScale
  animation mode : Subsystem
  elapsed track : Subsystem
  Out1 : Outport
  wires:
  Switch/1 -> Product/1
  WalkingScale/1 -> Switch/3
  RunningScale/1 -> Switch/1
  elapsed track/1(s) -> Product/2  "Time"
  Product/1 -> Bus Creator/2  "Time"
  Mux/1 -> elapsed track/1(vel), animation mode/1(vel)
  Bus Selector/1 -> Mux/1  "<VelocityX>"
  Bus Selector/2 -> Mux/2  "<VelocityY>"
  Bus Selector/3 -> Mux/3  "<VelocityZ>"
  animation mode/1(mode) -> Switch/2, Data Type Conversion/1
  In1/1 -> Bus Selector/1
  Bus Creator/1 -> Out1/1
  Data Type Conversion/1 -> Bus Creator/1  "Index"

== system TSR_Scenario_003_cs/Female_RegularAni_1/Dynamics_Empty ==
  note: For state mode 'Dynamic' positions
      | are not taken into account, as they
      | are computed by integrating velocity.
      | Click annotation for Help.
  note: For state mode 'Dynamic' positions
      | are not taken into account, as they
      | are computed by integrating velocity.
      | Click annotation for Help.
  Ground_{1..9} (9 alike) : Ground
  MuxState : Subsystem  Tag=mux/State  mask(Empty Dynamics State Block){positioningmode=on, TimeStep=1/100}
      mask prompts: positioningmode "Positioning Mode"; TimeStep "Auto Assigned: Time Step [s]"
      mask help:
      | Build the state of an actor based on user input.
      | The user can either use positioning mode or dynamics mode.
      | - When using positioning mode the position and orientation of the actor are set directly based on the input. Expected input is relative to the initial position and orientation of the actor. It's also possible to specify the velocity of the actor, though this input isn't used, only passed on.
      | - When using dynamics mode the position input is ignored. Expected input is velocity and orientation. The velocity is relative the current orientation of the actor, while orientation is relative to its initial orientation. The position of the actor is calculated based on the velocity and orientation given.
      settings: DeleteFcn=PreScanBlockDeleteFcn;
  STATE_Female_RegularAni_1 : Subsystem  Tag=mux/StatePort  Priority=0  LoadFcn=load PrescanStateActuatorData  mask(PreScan Sink Block: State){x0=TSR_Scenario_003_cs_cb1c89dfd10871a1, y0=TSR_Scenario_003_cs_b0d37aeb2aa747ff, z0=TSR_Scenario_003_cs_38ccddae174883be, Roll0=TSR_Scenario_003_cs_382e41ab6806a13f, Pitch0=TSR_Scenario_003_cs_68379cf1a8816ef6, Yaw0=TSR_Scenario_003_cs_c9d8e190789a4914, TimeStep=1/100}
      mask prompts: x0 "Ini x-position VEHICLE wrt GLOBAL axis system [m]"; y0 "Ini y-position VEHICLE wrt GLOBAL axis system [m]"; z0 "Ini z-position VEHICLE wrt GLOBAL axis system [m]"; Roll0 "Ini roll-angle BODY wrt VEHICLE axis system [deg]"; Pitch0 "Ini pitch-angle BODY wrt VEHICLE axis system [deg]"; Yaw0 "Ini yaw-angle VEHICLE wrt GLOBAL axis system [deg]"; TimeStep "Auto-Assigned: Upload Period [s]"
      mask help:
      | The Actor State contains a vector signal of size (9x1), containing the following signals:
      |
      | -  Position                  (x,y,z)                                     [m]
      | -  Velocity                  (vx,vy,vz)                               [m/s]
      | -  Angles                    (Roll, Pitch, Yaw)                   [rad]
      |
      | The Actor state is defined in the global axis system.
      | The state is superponed on the Initial position defined in the GUI.
      |
      | For more information, please click Help.
      settings: DeleteFcn=PreScanBlockDeleteFcn;
      mask Help: eval('openHelp(222)')
      mask Display: image(imread('State.png'))
  State : Outport  Tag=outport/StateOutport  SampleTime=1/100
  wires:
  STATE_Female_RegularAni_1/1(StateBus) -> State/1
  MuxState/1(state) -> STATE_Female_RegularAni_1/1(State)
  Ground_1/1 -> MuxState/1(x [m])
  Ground_2/1 -> MuxState/2(y [m])
  Ground_3/1 -> MuxState/3(z [m])
  Ground_4/1 -> MuxState/4(dx [m/s])
  Ground_5/1 -> MuxState/5(dy [m/s])
  Ground_6/1 -> MuxState/6(dz [m/s])
  Ground_7/1 -> MuxState/7(R [rad])
  Ground_8/1 -> MuxState/8(P [rad])
  Ground_9/1 -> MuxState/9(Y [rad])

== system TSR_Scenario_003_cs/Female_RegularAni_1/SELF_Demux ==
  SELF : Inport  OutDataTypeStr=Bus: PRESCAN_SELFSENSORDATA
  Bus Selector : BusSelector  OutputSignals=PositionX,PositionY,PositionZ,OrientationRoll,OrientationPitch,OrientationYaw,Velocity,Yaw_rate,Lat,Long,Alt
  Demux2 : Demux  Outputs=3
  Gain : Gain  Gain=180/pi
  Gain1 : Gain  Gain=180/pi
  Vector Concatenate1 : Concatenate  NumInputs=3
  compas converter : Subsystem
  x [m] : Outport
  y [m] : Outport  Port=2
  z [m] : Outport  Port=3
  rotx [deg] : Outport  Port=4
  roty [deg] : Outport  Port=5
  rotz [deg] : Outport  Port=6
  GPS lat [deg] : Outport  Port=7
  GPS long [deg] : Outport  Port=8
  GPS alt [m] : Outport  Port=9
  velocity [m/s] : Outport  Port=10
  heading [deg] : Outport  Port=11
  yaw rate [deg/s] : Outport  Port=12
  wires:
  Bus Selector/11 -> GPS alt [m]/1  "<Alt>"
  Bus Selector/10 -> GPS long [deg]/1  "<Long>"
  Bus Selector/9 -> GPS lat [deg]/1  "<Lat>"
  Bus Selector/8 -> Gain1/1  "<Yaw_rate>"
  Bus Selector/7 -> velocity [m/s]/1  "<Velocity>"
  Bus Selector/6 -> compas converter/1(rotz [rad]), Vector Concatenate1/3  "<OrientationYaw>"
  Bus Selector/5 -> Vector Concatenate1/2  "<OrientationPitch>"
  Bus Selector/4 -> Vector Concatenate1/1  "<OrientationRoll>"
  Vector Concatenate1/1 -> Gain/1
  Bus Selector/3 -> z [m]/1  "<PositionZ>"
  Bus Selector/2 -> y [m]/1  "<PositionY>"
  Bus Selector/1 -> x [m]/1  "<PositionX>"
  SELF/1 -> Bus Selector/1
  Gain/1 -> Demux2/1
  Demux2/1 -> rotx [deg]/1
  Demux2/2 -> roty [deg]/1
  Demux2/3 -> rotz [deg]/1
  compas converter/1(heading [deg]) -> heading [deg]/1
  Gain1/1 -> yaw rate [deg/s]/1

== system TSR_Scenario_003_cs/Female_RegularAni_1/VISUColorRegion_Lower_Body_Mux ==
  RGB [-,-,-] : Inport
  Bus Creator : BusCreator  OutDataTypeStr=Bus: PRESCAN_COLOR_DATA  NonVirtualBus=on
  Constant : Constant  Value=255  OutDataTypeStr=uint8
  Data Type Conversion : DataTypeConversion  OutDataTypeStr=uint8
  Data Type Conversion1 : DataTypeConversion  OutDataTypeStr=uint8
  Data Type Conversion2 : DataTypeConversion  OutDataTypeStr=uint8
  Demux : Demux  Outputs=3
  ColorRegion : Outport  OutDataTypeStr=Bus: PRESCAN_COLOR_DATA  PortDimensions=1
  wires:
  Constant/1 -> Bus Creator/4  "A"
  Data Type Conversion2/1 -> Bus Creator/3  "B"
  Data Type Conversion1/1 -> Bus Creator/2  "G"
  Data Type Conversion/1 -> Bus Creator/1  "R"
  Demux/3 -> Data Type Conversion2/1  "B"
  Demux/2 -> Data Type Conversion1/1  "G"
  Demux/1 -> Data Type Conversion/1  "R"
  RGB [-,-,-]/1 -> Demux/1
  Bus Creator/1 -> ColorRegion/1

== system TSR_Scenario_003_cs/Female_RegularAni_1/VISUColorRegion_Shoes_Mux ==
  RGB [-,-,-] : Inport
  Bus Creator : BusCreator  OutDataTypeStr=Bus: PRESCAN_COLOR_DATA  NonVirtualBus=on
  Constant : Constant  Value=255  OutDataTypeStr=uint8
  Data Type Conversion : DataTypeConversion  OutDataTypeStr=uint8
  Data Type Conversion1 : DataTypeConversion  OutDataTypeStr=uint8
  Data Type Conversion2 : DataTypeConversion  OutDataTypeStr=uint8
  Demux : Demux  Outputs=3
  ColorRegion : Outport  OutDataTypeStr=Bus: PRESCAN_COLOR_DATA  PortDimensions=1
  wires:
  Constant/1 -> Bus Creator/4  "A"
  Data Type Conversion2/1 -> Bus Creator/3  "B"
  Data Type Conversion1/1 -> Bus Creator/2  "G"
  Data Type Conversion/1 -> Bus Creator/1  "R"
  Demux/3 -> Data Type Conversion2/1  "B"
  Demux/2 -> Data Type Conversion1/1  "G"
  Demux/1 -> Data Type Conversion/1  "R"
  RGB [-,-,-]/1 -> Demux/1
  Bus Creator/1 -> ColorRegion/1

== system TSR_Scenario_003_cs/Female_RegularAni_1/VISUColorRegion_Upper_Body_Mux ==
  RGB [-,-,-] : Inport
  Bus Creator : BusCreator  OutDataTypeStr=Bus: PRESCAN_COLOR_DATA  NonVirtualBus=on
  Constant : Constant  Value=255  OutDataTypeStr=uint8
  Data Type Conversion : DataTypeConversion  OutDataTypeStr=uint8
  Data Type Conversion1 : DataTypeConversion  OutDataTypeStr=uint8
  Data Type Conversion2 : DataTypeConversion  OutDataTypeStr=uint8
  Demux : Demux  Outputs=3
  ColorRegion : Outport  OutDataTypeStr=Bus: PRESCAN_COLOR_DATA  PortDimensions=1
  wires:
  Constant/1 -> Bus Creator/4  "A"
  Data Type Conversion2/1 -> Bus Creator/3  "B"
  Data Type Conversion1/1 -> Bus Creator/2  "G"
  Data Type Conversion/1 -> Bus Creator/1  "R"
  Demux/3 -> Data Type Conversion2/1  "B"
  Demux/2 -> Data Type Conversion1/1  "G"
  Demux/1 -> Data Type Conversion/1  "R"
  RGB [-,-,-]/1 -> Demux/1
  Bus Creator/1 -> ColorRegion/1

== system TSR_Scenario_003_cs/Female_Regular_wBuggy_1/Animation ==
  In1 : Inport
  Bus Creator : BusCreator  Inputs=2  OutDataTypeStr=Bus: PRESCAN_ANIMACTUATORDATA  NonVirtualBus=on
  Bus Selector : BusSelector  OutputSignals=VelocityX,VelocityY,VelocityZ
  Mux : Mux  Inputs=3
  animation mode : Subsystem
  elapsed track : Subsystem
  Out1 : Outport
  wires:
  animation mode/1(mode) -> Bus Creator/1  "Index"
  Bus Creator/1 -> Out1/1
  In1/1 -> Bus Selector/1
  elapsed track/1(s) -> Bus Creator/2  "Time"
  Bus Selector/3 -> Mux/3  "<VelocityZ>"
  Bus Selector/2 -> Mux/2  "<VelocityY>"
  Bus Selector/1 -> Mux/1  "<VelocityX>"
  Mux/1 -> animation mode/1(vel), elapsed track/1(vel)

== system TSR_Scenario_003_cs/Female_Regular_wBuggy_1/Dynamics_Empty ==
  note: For state mode 'Dynamic' positions
      | are not taken into account, as they
      | are computed by integrating velocity.
      | Click annotation for Help.
  note: For state mode 'Dynamic' positions
      | are not taken into account, as they
      | are computed by integrating velocity.
      | Click annotation for Help.
  Ground_{1..9} (9 alike) : Ground
  MuxState : Subsystem  Tag=mux/State  mask(Empty Dynamics State Block){positioningmode=on, TimeStep=1/100}
      mask prompts: positioningmode "Positioning Mode"; TimeStep "Auto Assigned: Time Step [s]"
      mask help:
      | Build the state of an actor based on user input.
      | The user can either use positioning mode or dynamics mode.
      | - When using positioning mode the position and orientation of the actor are set directly based on the input. Expected input is relative to the initial position and orientation of the actor. It's also possible to specify the velocity of the actor, though this input isn't used, only passed on.
      | - When using dynamics mode the position input is ignored. Expected input is velocity and orientation. The velocity is relative the current orientation of the actor, while orientation is relative to its initial orientation. The position of the actor is calculated based on the velocity and orientation given.
      settings: DeleteFcn=PreScanBlockDeleteFcn;
  STATE_Female_Regular_wBuggy_1 : Subsystem  Tag=mux/StatePort  Priority=0  LoadFcn=load PrescanStateActuatorData  mask(PreScan Sink Block: State){x0=TSR_Scenario_003_cs_35d6077a5f3bdf8f, y0=TSR_Scenario_003_cs_1ea9b65b93b2d93e, z0=TSR_Scenario_003_cs_1f4a4c0163bc654f, Roll0=TSR_Scenario_003_cs_c1394d62e1abbae4, Pitch0=TSR_Scenario_003_cs_783b91f8e3e9acd3, Yaw0=TSR_Scenario_003_cs_f028791b9216ac63, TimeStep=1/100}
      mask prompts: x0 "Ini x-position VEHICLE wrt GLOBAL axis system [m]"; y0 "Ini y-position VEHICLE wrt GLOBAL axis system [m]"; z0 "Ini z-position VEHICLE wrt GLOBAL axis system [m]"; Roll0 "Ini roll-angle BODY wrt VEHICLE axis system [deg]"; Pitch0 "Ini pitch-angle BODY wrt VEHICLE axis system [deg]"; Yaw0 "Ini yaw-angle VEHICLE wrt GLOBAL axis system [deg]"; TimeStep "Auto-Assigned: Upload Period [s]"
      mask help:
      | The Actor State contains a vector signal of size (9x1), containing the following signals:
      |
      | -  Position                  (x,y,z)                                     [m]
      | -  Velocity                  (vx,vy,vz)                               [m/s]
      | -  Angles                    (Roll, Pitch, Yaw)                   [rad]
      |
      | The Actor state is defined in the global axis system.
      | The state is superponed on the Initial position defined in the GUI.
      |
      | For more information, please click Help.
      settings: DeleteFcn=PreScanBlockDeleteFcn;
      mask Help: eval('openHelp(222)')
      mask Display: image(imread('State.png'))
  State : Outport  Tag=outport/StateOutport  SampleTime=1/100
  wires:
  STATE_Female_Regular_wBuggy_1/1(StateBus) -> State/1
  MuxState/1(state) -> STATE_Female_Regular_wBuggy_1/1(State)
  Ground_1/1 -> MuxState/1(x [m])
  Ground_2/1 -> MuxState/2(y [m])
  Ground_3/1 -> MuxState/3(z [m])
  Ground_4/1 -> MuxState/4(dx [m/s])
  Ground_5/1 -> MuxState/5(dy [m/s])
  Ground_6/1 -> MuxState/6(dz [m/s])
  Ground_7/1 -> MuxState/7(R [rad])
  Ground_8/1 -> MuxState/8(P [rad])
  Ground_9/1 -> MuxState/9(Y [rad])
